simulink subsystem "rmsLimit"  (R2023b)
settings: Solver=VariableStepAuto  StartTime=0.0  StopTime=10.0  RelTol=1e-3
libraries: simulink x1
settings Model: Creator=jadam  LastModifiedBy=Veimar
settings DebuggingCC: UnconnectedInputMsg=warning  UnconnectedOutputMsg=warning  UnconnectedLineMsg=warning
settings ModelReferenceCC: EnableRefExpFcnMdlSchedulingChecks=on
settings RTWCC: DLArmComputeVersion=19.05

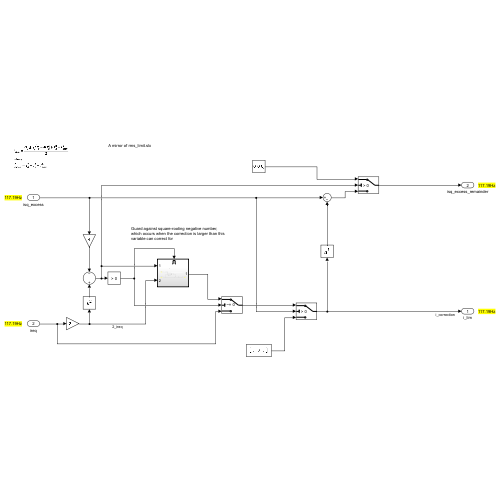
[thumbnail: Simulink's stored preview of the top-level diagram]
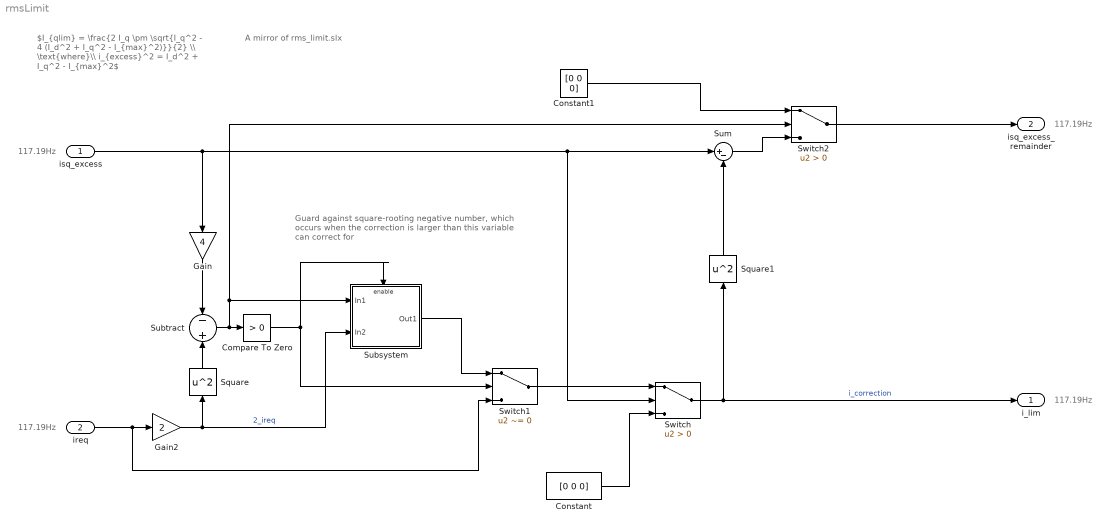
== system rmsLimit ==
  note: A mirror of rms_limit.slx
  note: $I_{qlim} = \frac{2 I_q \pm \sqrt{I_q^2 - 4 (I_d^2 + I_q^2 - I_{max}^2)}}{2} \\ \text{where}\\ i_{excess}^2 = I_d^2 + I_q^2 - I_{max}^2$
  note: Guard against square-rooting negative number,
      | which occurs when the correction is larger than this
      | variable can correct for
  note: 117.19Hz
  note: 117.19Hz
  note: 117.19Hz
  note: 117.19Hz
  isq_excess : Inport  OutDataTypeStr=single  PortDimensions=3
  ireq : Inport  Port=2  OutDataTypeStr=single  PortDimensions=3
  Compare To Zero : simulink/Logic and Bit Operations/Compare To Zero  relop=>  OutDataTypeStr=boolean
  Constant : Constant  Value=[0 0 0]  OutDataTypeStr=single
  Constant1 : Constant  Value=[0 0 0]  OutDataTypeStr=single
  Gain : Gain  Gain=4
  Gain2 : Gain  Gain=2  ParamDataTypeStr=single  OutDataTypeStr=single
  Square : Math  Operator=square
  Square1 : Math  Operator=square
  Subsystem : Subsystem
  Subtract : Sum  Inputs=-|+
  Sum : Sum  Inputs=|+-
  Switch : Switch  Criteria=u2 > Threshold  SaturateOnIntegerOverflow=off  InputSameDT=off
  Switch1 : Switch  Criteria=u2 ~= 0  SaturateOnIntegerOverflow=off  InputSameDT=off
  Switch2 : Switch  Criteria=u2 > Threshold  SaturateOnIntegerOverflow=off  InputSameDT=off
  i_lim : Outport  OutDataTypeStr=single  PortDimensions=3
  isq_excess_remainder : Outport  Port=2  OutDataTypeStr=single  PortDimensions=3
  wires:
  isq_excess/1 -> Gain/1, Switch/2, Sum/1
  Constant/1 -> Switch/3
  Switch/1 -> i_lim/1, Square1/1  "i_correction"
  Switch1/1 -> Switch/1
  ireq/1 -> Gain2/1, Switch1/3
  Gain/1 -> Subtract/1
  Subtract/1 -> Compare To Zero/1, Subsystem/1(In1), Switch2/2
  Compare To Zero/1 -> Switch1/2, Subsystem/Enable
  Square/1 -> Subtract/2
  Gain2/1 -> Square/1, Subsystem/2(In2)  "2_ireq"
  Subsystem/1(Out1) -> Switch1/1
  Constant1/1 -> Switch2/1
  Sum/1 -> Switch2/3
  Square1/1 -> Sum/2
  Switch2/1 -> isq_excess_remainder/1

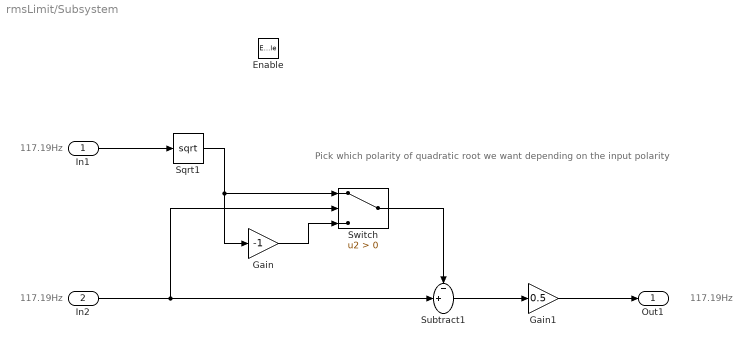
== system rmsLimit/Subsystem ==
  note: 117.19Hz
  note: 117.19Hz
  note: 117.19Hz
  note: Pick which polarity of quadratic root we want depending on the input polarity
  In1 : Inport
  In2 : Inport  Port=2
  Enable : EnablePort  StatesWhenEnabling=reset
  Gain : Gain  Gain=-1
  Gain1 : Gain  Gain=0.5
  Sqrt1 : Sqrt  OutputSignalType=real
  Subtract1 : Sum  Inputs=-+|
  Switch : Switch  Criteria=u2 > Threshold  SaturateOnIntegerOverflow=off  InputSameDT=off
  Out1 : Outport  OutputWhenDisabled=reset  InitialOutput=0
  wires:
  Switch/1 -> Subtract1/1
  Gain/1 -> Switch/3
  Sqrt1/1 -> Gain/1, Switch/1
  In1/1 -> Sqrt1/1
  Subtract1/1 -> Gain1/1
  In2/1 -> Subtract1/2, Switch/2
  Gain1/1 -> Out1/1
